simulink model "SensorFusionTest"  (R2016b)
settings: Solver=VariableStepAuto  StartTime=0.0  StopTime=20.0  RelTol=1e-3
undefined symbols (not defined in the file): aMean, aVar, gVar, mMean, mVar
libraries: quadLibrary x6
settings Model: DataDictionary=quadCopterDD.sldd  Creator=nikol  LastModifiedBy=nikol
settings DebuggingCC: ParameterPrecisionLossMsg=none

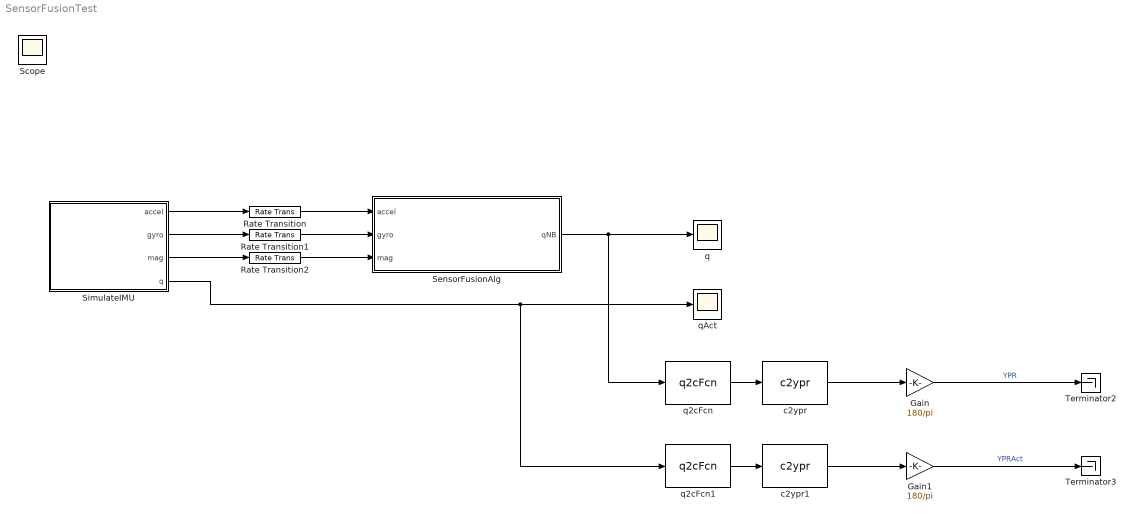
== system SensorFusionTest ==
  Gain : Gain  Gain=180/pi
  Gain1 : Gain  Gain=180/pi
  Rate Transition : RateTransition  Deterministic=off  OutPortSampleTime=1/200
  Rate Transition1 : RateTransition  Deterministic=off  OutPortSampleTime=1/200
  Rate Transition2 : RateTransition  Deterministic=off  OutPortSampleTime=1/200
  SensorFusionAlg : Subsystem  TreatAsAtomicUnit=on
  SimulateIMU : Subsystem  TreatAsAtomicUnit=on
  Terminator2 : Terminator
  Terminator3 : Terminator
  c2ypr : quadLibrary/c2ypr
  c2ypr1 : quadLibrary/c2ypr
  q : Scope
  q2cFcn : quadLibrary/q2cFcn
  q2cFcn1 : quadLibrary/q2cFcn
  qAct : Scope
  Scope : Scope
  wires:
  SimulateIMU/3(mag) -> Rate Transition2/1
  SimulateIMU/2(gyro) -> Rate Transition1/1
  SimulateIMU/1(accel) -> Rate Transition/1
  Rate Transition/1 -> SensorFusionAlg/1(accel)
  Rate Transition1/1 -> SensorFusionAlg/2(gyro)
  Rate Transition2/1 -> SensorFusionAlg/3(mag)
  SensorFusionAlg/1(qNB) -> q2cFcn/1, q/1
  SimulateIMU/4(q) -> q2cFcn1/1, qAct/1
  q2cFcn/1 -> c2ypr/1
  q2cFcn1/1 -> c2ypr1/1
  Gain/1 -> Terminator2/1  "YPR"
  Gain1/1 -> Terminator3/1  "YPRAct"
  c2ypr/1 -> Gain/1
  c2ypr1/1 -> Gain1/1

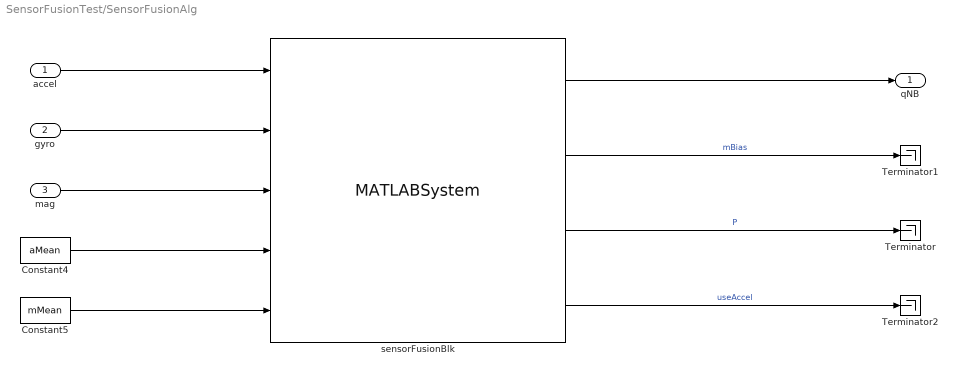
== system SensorFusionTest/SensorFusionAlg ==
  accel : Inport
  gyro : Inport  Port=2
  mag : Inport  Port=3
  Constant4 : Constant  Value=aMean  OutDataTypeStr=single
  Constant5 : Constant  Value=mMean  OutDataTypeStr=single
  Terminator : Terminator
  Terminator1 : Terminator
  Terminator2 : Terminator
  sensorFusionBlk : MATLABSystem  System=sensorFusionEKFSysObj  Avar=aVar  AvarDisable=single([1 1 1]*1e4)  accelMagDevThresh=single(0.1)  Mvar=mVar  Gvar=gVar  MagScaleFactor=single(100)  Pinit=Pinit  Ts=single(1/200)  SimulateUsing=Interpreted execution
      mask Type: sensorFusionEKFSysObj
      mask Display:
      | disp('sensorFusionEKFSysObj');
      | port_label('input',1,'a');
      | port_label('input',2,'w');
      | port_label('input',3,'m');
      | port_label('input',4,'g');
      | port_label('input',5,'h');
      | port_label('output',1,'qNB');
      | port_label('output',2,'mBias');
      | port_label('output',3,'P');
      | port_label('output',4,'useAccel');
  qNB : Outport
  wires:
  gyro/1 -> sensorFusionBlk/2
  accel/1 -> sensorFusionBlk/1
  Constant4/1 -> sensorFusionBlk/4
  sensorFusionBlk/1 -> qNB/1
  sensorFusionBlk/2 -> Terminator1/1  "mBias"
  Constant5/1 -> sensorFusionBlk/5
  mag/1 -> sensorFusionBlk/3
  sensorFusionBlk/3 -> Terminator/1  "P"
  sensorFusionBlk/4 -> Terminator2/1  "useAccel"

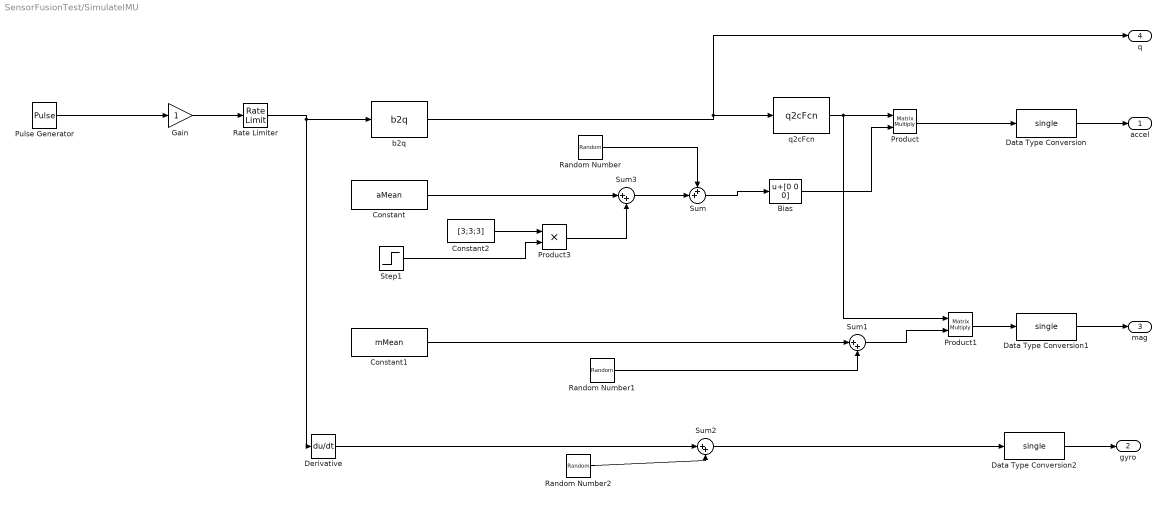
== system SensorFusionTest/SimulateIMU ==
  Bias : Bias  Bias=[0 0 0]
  Constant : Constant  Value=aMean
  Constant1 : Constant  Value=mMean
  Constant2 : Constant  Value=[3;3;3]
  Data Type Conversion : DataTypeConversion  OutDataTypeStr=single
  Data Type Conversion1 : DataTypeConversion  OutDataTypeStr=single
  Data Type Conversion2 : DataTypeConversion  OutDataTypeStr=single
  Derivative : Derivative
  Gain : Gain
  Product : Product  Multiplication=Matrix(*)
  Product1 : Product  Multiplication=Matrix(*)
  Product3 : Product
  Pulse Generator : DiscretePulseGenerator  PulseType=Time based  Period=10  PulseWidth=5  PhaseDelay=[1 3 5]
  Random Number : RandomNumber  Variance=aVar  SampleTime=1/1000
  Random Number1 : RandomNumber  Variance=mVar  SampleTime=1/1000
  Random Number2 : RandomNumber  Variance=gVar  SampleTime=1/1000
  Rate Limiter : RateLimiter  RisingSlewLimit=180*pi/180  FallingSlewLimit=-180*pi/180  SampleTimeMode=inherited
  Step1 : Step  Time=15  After=0  SampleTime=0
  Sum : Sum  Inputs=++|
  Sum1 : Sum  Inputs=|++
  Sum2 : Sum  Inputs=|++
  Sum3 : Sum  Inputs=|++
  b2q : quadLibrary/b2q
  q2cFcn : quadLibrary/q2cFcn
  accel : Outport
  gyro : Outport  Port=2
  mag : Outport  Port=3
  q : Outport  Port=4
  wires:
  b2q/1 -> q/1, q2cFcn/1
  q2cFcn/1 -> Product1/1, Product/1
  Constant/1 -> Sum3/1
  Product/1 -> Data Type Conversion/1
  Product1/1 -> Data Type Conversion1/1
  Derivative/1 -> Sum2/1
  Rate Limiter/1 -> b2q/1, Derivative/1
  Data Type Conversion/1 -> accel/1
  Data Type Conversion1/1 -> mag/1
  Data Type Conversion2/1 -> gyro/1
  Bias/1 -> Product/2
  Sum/1 -> Bias/1
  Random Number/1 -> Sum/1
  Random Number1/1 -> Sum1/2
  Sum1/1 -> Product1/2
  Random Number2/1 -> Sum2/2
  Constant1/1 -> Sum1/1
  Sum2/1 -> Data Type Conversion2/1
  Gain/1 -> Rate Limiter/1
  Pulse Generator/1 -> Gain/1
  Step1/1 -> Product3/2
  Product3/1 -> Sum3/2
  Sum3/1 -> Sum/2
  Constant2/1 -> Product3/1
